simulink model "hbridge_inverter_lc_open_loop"  (R2025b)
settings: Solver=ode3  StartTime=0.0  StopTime=0.1  FixedStep=1e-06  RelTol=1e-3
values from neighbouring files (symbols this model uses):
  lc_tf_den = [      L_f * C_f * (R_load + R_d_total),      L_f + R_Lf * C_f * (R_load + R_d_total) + R_load * C_f * R_d_total,      R_Lf + R_load  ]    [inverter_params.m]
  lc_tf_num = [R_load * C_f * R_d_total, R_load]    [inverter_params.m]
  m_a = 0.85    [inverter_params.m]
  omega_0 = 2 * pi * f_grid    (= 314.159265359)    [inverter_params.m]
  R_load = (V_ac_rms^2) / P_nom    [inverter_params.m]
  Vdc = 48.0    (= 48)    [inverter_params.m]
libraries: simulink x1
settings Model: Creator=hemanggadhvi  LastModifiedBy=hemanggadhvi

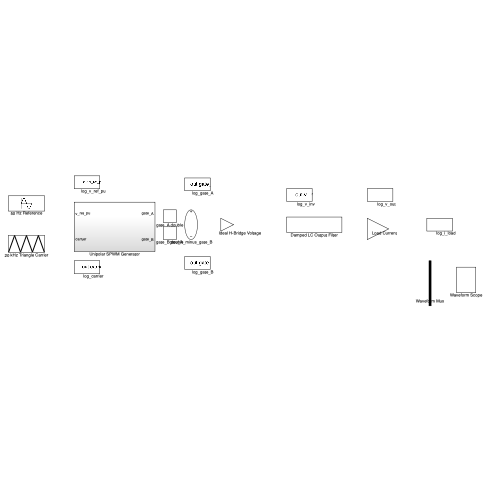
[thumbnail: Simulink's stored preview of the top-level diagram]
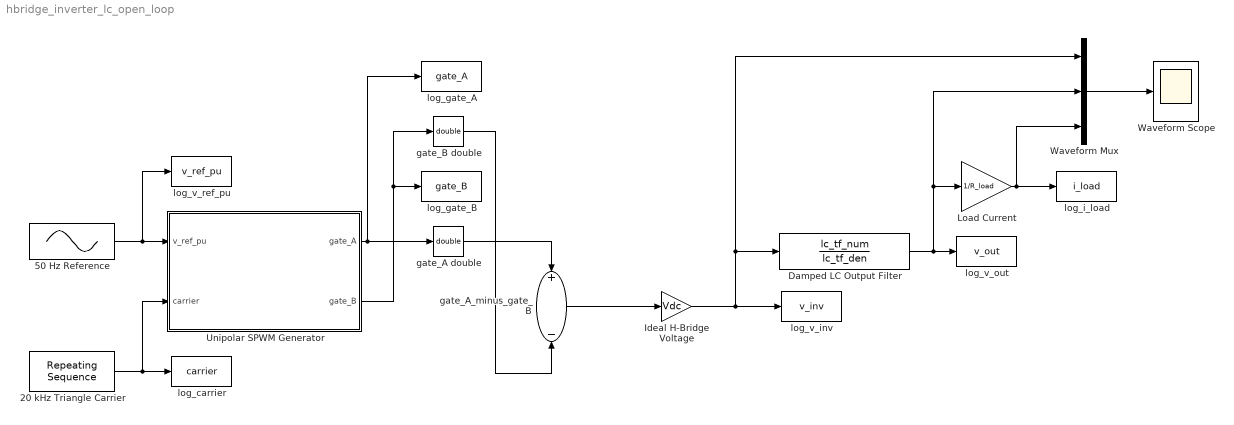
== system hbridge_inverter_lc_open_loop ==
  20 kHz Triangle Carrier : simulink/Sources/Repeating Sequence  rep_seq_t=carrier_time  rep_seq_y=carrier_values
  50 Hz Reference : Sin  Amplitude=m_a  Frequency=omega_0  SampleTime=0
  Damped LC Output Filter : TransferFcn  Numerator=lc_tf_num  Denominator=lc_tf_den
  Ideal H-Bridge Voltage : Gain  Gain=Vdc
  Load Current : Gain  Gain=1/R_load
  Unipolar SPWM Generator : Subsystem
  Waveform Mux : Mux  Inputs=3
  Waveform Scope : Scope
  gate_A double : DataTypeConversion  OutDataTypeStr=double  SaturateOnIntegerOverflow=off  RndMeth=Floor
  gate_A_minus_gate_B : Sum  Inputs=+-
  gate_B double : DataTypeConversion  OutDataTypeStr=double  SaturateOnIntegerOverflow=off  RndMeth=Floor
  log_carrier : ToWorkspace  VariableName=carrier  SaveFormat=Timeseries  SampleTime=-1
  log_gate_A : ToWorkspace  VariableName=gate_A  SaveFormat=Timeseries  SampleTime=-1
  log_gate_B : ToWorkspace  VariableName=gate_B  SaveFormat=Timeseries  SampleTime=-1
  log_i_load : ToWorkspace  VariableName=i_load  SaveFormat=Timeseries  SampleTime=-1
  log_v_inv : ToWorkspace  VariableName=v_inv  SaveFormat=Timeseries  SampleTime=-1
  log_v_out : ToWorkspace  VariableName=v_out  SaveFormat=Timeseries  SampleTime=-1
  log_v_ref_pu : ToWorkspace  VariableName=v_ref_pu  SaveFormat=Timeseries  SampleTime=-1
  wires:
  Waveform Mux/1 -> Waveform Scope/1
  Damped LC Output Filter/1 -> Load Current/1, Waveform Mux/2, log_v_out/1
  Ideal H-Bridge Voltage/1 -> Waveform Mux/1, Damped LC Output Filter/1, log_v_inv/1
  Load Current/1 -> Waveform Mux/3, log_i_load/1
  gate_A_minus_gate_B/1 -> Ideal H-Bridge Voltage/1
  gate_A double/1 -> gate_A_minus_gate_B/1
  gate_B double/1 -> gate_A_minus_gate_B/2
  Unipolar SPWM Generator/2(gate_B) -> log_gate_B/1, gate_B double/1
  Unipolar SPWM Generator/1(gate_A) -> log_gate_A/1, gate_A double/1
  20 kHz Triangle Carrier/1 -> log_carrier/1, Unipolar SPWM Generator/2(carrier)
  50 Hz Reference/1 -> log_v_ref_pu/1, Unipolar SPWM Generator/1(v_ref_pu)

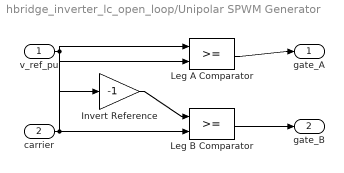
== system hbridge_inverter_lc_open_loop/Unipolar SPWM Generator ==
  v_ref_pu : Inport
  carrier : Inport  Port=2
  Invert Reference : Gain  Gain=-1
  Leg A Comparator : RelationalOperator  OutDataTypeStr=boolean  RndMeth=Simplest  InputSameDT=off
  Leg B Comparator : RelationalOperator  OutDataTypeStr=boolean  RndMeth=Simplest  InputSameDT=off
  gate_A : Outport
  gate_B : Outport  Port=2
  wires:
  v_ref_pu/1 -> Leg A Comparator/1, Invert Reference/1
  carrier/1 -> Leg A Comparator/2, Leg B Comparator/2
  Invert Reference/1 -> Leg B Comparator/1
  Leg A Comparator/1 -> gate_A/1
  Leg B Comparator/1 -> gate_B/1
